simulink subsystem "ControlObject"  (R2023a)
settings: Solver=VariableStepAuto  StartTime=0.0  StopTime=10.0  RelTol=1e-3
model mask{Ku=7.27, V=24, R=10, n0=14400, I0=60 * 10^(-3), Kw=600, Km=16 * 10^(-3), L=350 * 10^(-6), Jr=500 * 10^(-9), Kf=0.01, Jred=2.4, ired=100, Kfred=0.002, Jrp=1, irp=20, Kfrp=0.001, Kisens=0.001, KangleSens=2, KspeedSens=0.2, M_st=0.1, M_p=0.2, KerL=1, g=9.81}
  mask prompts: Ku "Power gain coefficient"; V "Nominal Voltage"; R "Resistance"; n0 "Nominal speed"; I0 "Nominal current"; Kw "Speed constant"; Km "Torque constant"; L "Inductivity"; Jr "Rotor inertia"; Kf "Friction coefficient"; Jred "Inertia"; ired "Transfer coefficient"; Kfred "Friction corfficient"; Jrp "Inertia"; irp "Transfer coefficient"; Kfrp "Friction coefficient"; Kisens "Current coefficient"; KangleSens "Angle coefficient"; KspeedSens "Speed coefficient"; M_st "Kernel mass"; M_p "Basement mass"; KerL "Kernel length"
settings Model: Creator=user  LastModifiedBy=User

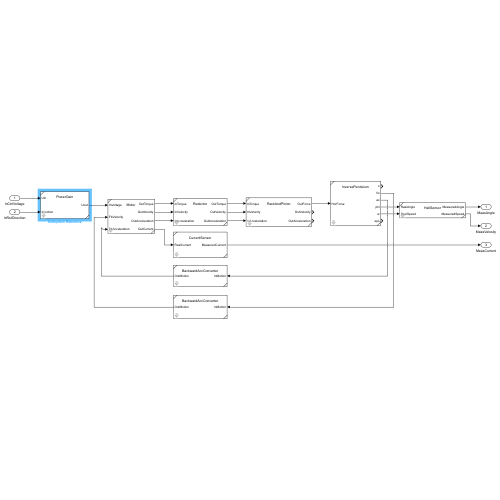
[thumbnail: Simulink's stored preview of the top-level diagram]
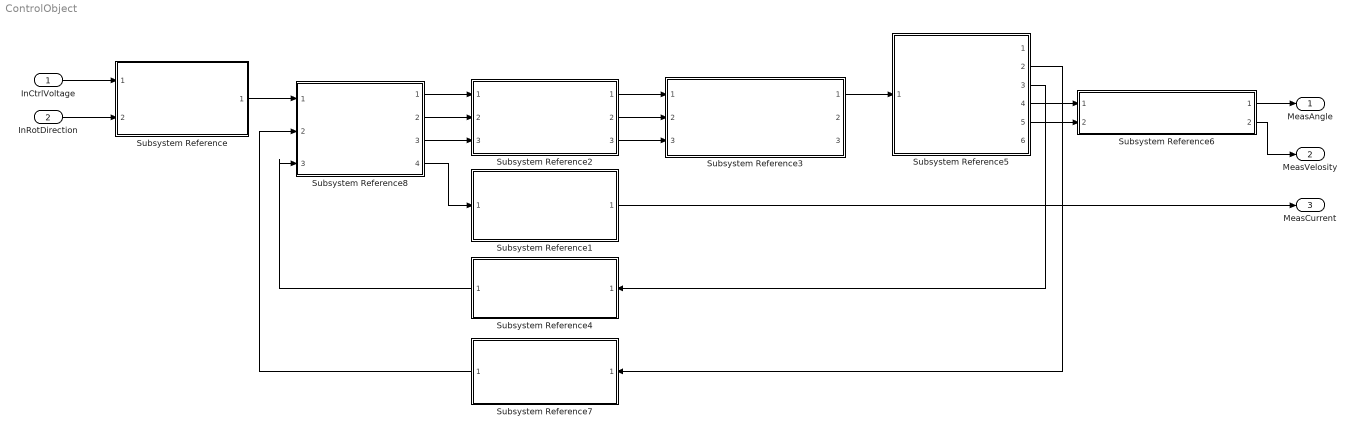
== system ControlObject ==
  InCtrlVoltage : Inport
  InRotDirection : Inport  Port=2
  Subsystem Reference : Subsystem  ReferencedSubsystem=PowerGain  Ku=Ku
  Subsystem Reference1 : Subsystem  ReferencedSubsystem=CurrentSensor  Ku=Kisens
  Subsystem Reference2 : Subsystem  ReferencedSubsystem=Reductor  J_gear=Jred  i_gear=ired  vis_friction_coef_gear=Kfred
  Subsystem Reference3 : Subsystem  ReferencedSubsystem=RackAndPinion  i_gear=Jrp  J_gear=irp  Friction_coeff_gear=Kfrp
  Subsystem Reference4 : Subsystem  ReferencedSubsystem=BackwardAccConverter  i_RackAndPinion=irp  i_Gearbox=ired
  Subsystem Reference5 : Subsystem  ReferencedSubsystem=InversePendulum  M_p=M_p  m_st=M_st  l=KerL  g=g
  Subsystem Reference6 : Subsystem  ReferencedSubsystem=HallSensor  speed_coef=KspeedSens  angle_coef=KangleSens
  Subsystem Reference7 : Subsystem  ReferencedSubsystem=BackwardAccConverter  i_RackAndPinion=irp  i_Gearbox=ired
  Subsystem Reference8 : Subsystem  ReferencedSubsystem=Motor  Un=V  R=R  Ni=n0  Ii=I0  Kn=Kw  Km=Km  L=L  J_motor=Jr  vis_friction_coef_motor=Kf
  MeasAngle : Outport
  MeasVelosity : Outport  Port=2
  MeasCurrent : Outport  Port=3
  wires:
  InCtrlVoltage/1 -> Subsystem Reference/1
  InRotDirection/1 -> Subsystem Reference/2
  Subsystem Reference2/1 -> Subsystem Reference3/1
  Subsystem Reference2/2 -> Subsystem Reference3/2
  Subsystem Reference2/3 -> Subsystem Reference3/3
  Subsystem Reference3/1 -> Subsystem Reference5/1
  Subsystem Reference1/1 -> MeasCurrent/1
  Subsystem Reference8/1 -> Subsystem Reference2/1
  Subsystem Reference8/2 -> Subsystem Reference2/2
  Subsystem Reference8/3 -> Subsystem Reference2/3
  Subsystem Reference/1 -> Subsystem Reference8/1
  Subsystem Reference8/4 -> Subsystem Reference1/1
  Subsystem Reference5/5 -> Subsystem Reference6/2
  Subsystem Reference5/4 -> Subsystem Reference6/1
  Subsystem Reference6/2 -> MeasVelosity/1
  Subsystem Reference6/1 -> MeasAngle/1
  Subsystem Reference7/1 -> Subsystem Reference8/2
  Subsystem Reference4/1 -> Subsystem Reference8/3
  Subsystem Reference5/3 -> Subsystem Reference4/1
  Subsystem Reference5/2 -> Subsystem Reference7/1
